simulink model "ctrl_PF"  (R2022b)
settings: Solver=FixedStepAuto  StartTime=0.0  StopTime=Tf  FixedStep=0.05  RelTol=1e-3
StopFcn:
  | save('testdata')
values from neighbouring files (symbols this model uses):
  Ba_0 = [0 0 0 0 0 0]    [run.m]    (also in testdata.mat)
  Bb = 4418825.3321    [testdata.mat]
  Bv_0 = [-5.14444 0 0 0 0 0]    [run.m]    (also in testdata.mat)
  Bx_0 = [-Cp(1,1) -Cp(2,1) Cp(3,1) 0 0 -pi]    [run.m]    (also in testdata.mat = [7.34788079488e-14 -400 -100 0 0 -3.14159265359])
  Cp = [x;y;z]    [run.m]    (also in testdata.mat = [-7.34788079488e-14 400 -100 -24.1026674607 399.273166418 -1)
  Cp_prime = Cp*Diff    [run.m]    (also in testdata.mat = [-4.77232815721 -0.143913049279 0 -4.75515990164 -0.42831409)
  d = 50    [run.m]    (also in testdata.mat)
  dA_BP1 = [0.00388591051125 0.00354364911083 0.00553040741788 0.00502167988714 0.0078585088908 0.00748424955325 0.0119232766011 0.0109054787122 0.0168329706434 0.016985509009 0.0156802934897 0.014556760782 ... (616 elements, 616x1)]    [testdata.mat]
  dA_BP2 = [0.00388594063171 0.00354357191533 0.00553040491113 0.00502170939051 0.00785855989083 0.00748435285791 0.0119232653011 0.0109054419481 0.0168329955973 0.0169854794658 0.015680230324 0.0145567225609 ... (616 elements, 616x1)]    [testdata.mat]
  dA_Hull = [0.896301676511 0.898896720864 0.884294141897 0.886832830172 0.870887902011 0.873360353662 0.856223658523 0.858613244346 0.840314828191 0.842595287849 0.823129385532 0.8253007603 ... (2914 elements, 2914x1)]    [testdata.mat]
  dA_PH = [0.00917454029683 0.00917454029683 0.00646521761836 0.00644666811643 0.011728531678 0.0107683420972 0.0165186720105 0.0100399866209 0.0121147162203 0.00917369783051 0.00917369783051 0.00646462373197 ... (550 elements, 550x1)]    [testdata.mat]
  dA_Sail = [0.08073747293 0.0655437895785 0.0678199581962 0.211496702297 0.185444652254 0.10949647106 0.0763960001413 0.0735864235671 0.0440728222699 0.281106392154 0.32735958292 0.104041938486 ... (564 elements, 564x1)]    [testdata.mat]
  dA_SProot = [0.0225345452169 0.0247277274893 0.0225345452169 0.0480467976325 0.0166447079844 0.0410754287554 0.0247277274893 0.0480467976325 0.0468898715351 0.0839833312794 0.0166447079844 0.0255016718 ... (904 elements, 904x1)]    [testdata.mat]
  dA_X1a = [0.0149621011817 0.0166706156701 0.0341149781095 0.0355915100668 0.0512235531199 0.0489176133683 0.0604458424392 0.0503279152264 0.0577124835488 0.0401555322121 0.044833653096 0.0251568218541 ... (200 elements, 200x1)]    [testdata.mat]
  dA_X1b = [0.0149621011817 0.0166706156701 0.0341149781095 0.0355915100668 0.0512235531199 0.0489176133683 0.0604458424392 0.0503279152264 0.0577124835488 0.0401555322121 0.044833653096 0.0251568218541 ... (200 elements, 200x1)]    [testdata.mat]
  dA_X2a = [0.0149620639393 0.0166705502855 0.0341150948266 0.0355913495849 0.051223110376 0.0489180393921 0.0604458270347 0.0503275686692 0.0577128112225 0.0401556683139 0.0448334591683 0.0251566482124 ... (200 elements, 200x1)]    [testdata.mat]
  dA_X2b = [0.0149620639393 0.0166705502855 0.0341150948266 0.0355913495849 0.051223110376 0.0489180393921 0.0604458270347 0.0503275686692 0.0577128112225 0.0401556683139 0.0448334591683 0.0251566482124 ... (200 elements, 200x1)]    [testdata.mat]
  dA_X3a = [0.0149621011817 0.0166706156701 0.0341149781095 0.0355915100668 0.0512235531199 0.0489176133683 0.0604458424392 0.0503279152264 0.0577124835488 0.0401555322121 0.044833653096 0.0251568218541 ... (200 elements, 200x1)]    [testdata.mat]
  dA_X3b = [0.0149621011817 0.0166706156701 0.0341149781095 0.0355915100668 0.0512235531199 0.0489176133683 0.0604458424392 0.0503279152264 0.0577124835488 0.0401555322121 0.044833653096 0.0251568218541 ... (200 elements, 200x1)]    [testdata.mat]
  dA_X4a = [0.0149621011817 0.0166706156701 0.0341149781095 0.0355915100668 0.0512235531199 0.0489176133683 0.0604458424392 0.0503279152264 0.0577124835488 0.0401555322121 0.044833653096 0.0251568218541 ... (200 elements, 200x1)]    [testdata.mat]
  dA_X4b = [0.0149621011817 0.0166706156701 0.0341149781095 0.0355915100668 0.0512235531199 0.0489176133683 0.0604458424392 0.0503279152264 0.0577124835488 0.0401555322121 0.044833653096 0.0251568218541 ... (200 elements, 200x1)]    [testdata.mat]
  Ixx = 52300000    [testdata.mat]
  Ixy = 0    [testdata.mat]
  Ixz = 0    [testdata.mat]
  Iyy = 1375000000    [testdata.mat]
  Iyz = 0    [testdata.mat]
  Izz = 1367000000    [testdata.mat]
  Ky = 1    [run.m]    (also in testdata.mat)
  Mb = 4418825.3321    [testdata.mat]
  n_BP1 = [-0.7747315 -0.03638153 -0.4095958 0 -0.1221389 0 -0.01670914 0 0.005209626 0 0.03404154 0 ... (1848 elements, 616x3)]    [testdata.mat]
  n_BP2 = [-0.774731517 -0.0363815315 -0.409595788 0 -0.122138903 0 -0.0167091396 0 0.00520962616 0 0.0340415388 0 ... (1848 elements, 616x3)]    [testdata.mat]
  n_Hull = [-3.334458e-05 -1.700098e-14 -3.354233e-05 -1.686235e-14 -3.289162e-05 -1.685701e-14 -3.291391e-05 -1.698144e-14 -3.338145e-05 -1.688959e-14 -3.29289e-05 -1.682536e-14 ... (8742 elements, 2914x3)]    [testdata.mat]
  n_PH = [0 0 0.01711651 0.01711627 0.2676807 0.2676804 0.7675173 0.7675174 0.9857236 0 0 0.01711456 ... (1650 elements, 550x3)]    [testdata.mat]
  n_Sail = [-0.05126832 -0.05168081 -0.0485872 -0.03288998 -0.03203588 -0.04435105 -0.04335441 -0.04419429 -0.05169604 0.01094904 0.01649325 -0.03825178 ... (1692 elements, 564x3)]    [testdata.mat]
  n_SProot = [-0.7837688 -0.7969784 -0.7837688 -0.79448 -0.280412 -0.3378876 -0.7969784 -0.79448 -0.7910827 -0.3483897 -0.280412 -0.2790298 ... (2712 elements, 904x3)]    [testdata.mat]
  n_X2a = [-0.283297986 -0.283136904 -0.283195704 -0.28313759 -0.2831586 -0.283137113 -0.28313911 -0.283136606 -0.283121586 -0.283136815 -0.283108413 -0.283138901 ... (600 elements, 200x3)]    [testdata.mat]
  n_X2b = [-0.283297986 -0.283136904 -0.283195704 -0.28313759 -0.2831586 -0.283137113 -0.28313911 -0.283136606 -0.283121586 -0.283136815 -0.283108413 -0.283138901 ... (600 elements, 200x3)]    [testdata.mat]
  n_X3a = [-0.283298 -0.2831369 -0.2831957 -0.2831376 -0.2831586 -0.2831371 -0.2831391 -0.2831366 -0.2831216 -0.2831368 -0.2831084 -0.2831389 ... (600 elements, 200x3)]    [testdata.mat]
  n_X4a = [-0.283298 -0.2831369 -0.2831957 -0.2831376 -0.2831586 -0.2831371 -0.2831391 -0.2831366 -0.2831216 -0.2831368 -0.2831084 -0.2831389 ... (600 elements, 200x3)]    [testdata.mat]
  n_X4b = [-0.283298 -0.2831369 -0.2831957 -0.2831376 -0.2831586 -0.2831371 -0.2831391 -0.2831366 -0.2831216 -0.2831368 -0.2831084 -0.2831389 ... (600 elements, 200x3)]    [testdata.mat]
  nt_BP1 = 616    [testdata.mat]
  nt_BP2 = 616    [testdata.mat]
  nt_Hull = 2914    [testdata.mat]
  nt_PH = 550    [testdata.mat]
  nt_Sail = 564    [testdata.mat]
  nt_SProot = 904    [testdata.mat]
  nt_X1a = 200    [testdata.mat]
  nt_X1b = 200    [testdata.mat]
  nt_X2a = 200    [testdata.mat]
  nt_X2b = 200    [testdata.mat]
  nt_X3a = 200    [testdata.mat]
  nt_X3b = 200    [testdata.mat]
  nt_X4a = 200    [testdata.mat]
  nt_X4b = 200    [testdata.mat]
  Seastate = 0    [run.m]    (also in testdata.mat)
  Tf = 500    [run.m]    (also in testdata.mat)
  v_ref = Bv_0(1)    [run.m]    (also in testdata.mat = -5.14444)
  vt1_BP1 = [-11.0524049722 -10.9924120522 -10.9924120522 -10.8819663922 -10.8819663922 -10.7297166322 -10.7297166322 -10.5070632922 -10.5070632922 -10.1807245522 -10.1807245522 -9.8815181122 ... (1848 elements, 616x3)]    [testdata.mat]
  vt1_BP2 = [-11.0524048318 -10.9924111396 -10.9924111396 -10.8819658306 -10.8819658306 -10.7297157898 -10.7297157898 -10.5070637134 -10.5070637134 -10.1807238502 -10.1807238502 -9.8815188844 ... (1848 elements, 616x3)]    [testdata.mat]
  vt1_Hull = [3.5122487678 3.7304022878 5.2621803278 5.4863499878 6.9866994878 7.2167238278 8.6832650078 8.9189474678 10.3493567078 10.5904445678 11.9823842078 12.2286247478 ... (8742 elements, 2914x3)]    [testdata.mat]
  vt1_PH = [37.3342788278 37.3342788278 37.4268866678 37.4268866678 37.5892452278 37.5892452278 37.7549453078 37.7549453078 37.8074619278 37.3342788278 37.3342788278 37.4268866678 ... (1650 elements, 550x3)]    [testdata.mat]
  vt1_Sail = [-12.4909433722 -12.1578443722 -12.0399645322 -11.2138368922 -10.6240515922 -11.5111900522 -11.9364967522 -11.6561249722 -12.4909433722 -7.5732648922 -6.8453119522 -11.1890071522 ... (1692 elements, 564x3)]    [testdata.mat]
  vt1_SProot = [29.2099766678 29.1371231078 29.0494854278 29.2099766678 29.2862630078 29.4526510478 29.0494854278 29.1261368078 29.3369263478 29.5706712878 29.0494854278 29.3857364078 ... (2712 elements, 904x3)]    [testdata.mat]
  vt1_X1a = [29.3961751478 29.4776282078 29.4776282078 29.7060309278 29.7060309278 30.0693861278 30.0693861278 30.5458756478 30.5458756478 31.0830460478 31.0830460478 31.6023926678 ... (600 elements, 200x3)]    [testdata.mat]
  vt1_X1b = [29.6638337078 29.6638337078 29.9620713878 29.9620713878 30.3181187678 30.3181187678 30.7116389078 30.7116389078 31.1104380878 31.1104380878 31.4810519678 31.4810519678 ... (600 elements, 200x3)]    [testdata.mat]
  vt1_X2a = [29.3961767624 29.4776272952 29.4776272952 29.7060326828 29.7060326828 30.0693842324 30.0693842324 30.5458736822 30.5458736822 31.083047171 31.083047171 31.6023916148 ... (600 elements, 200x3)]    [testdata.mat]
  vt1_X2b = [29.6638345502 29.6638345502 29.9620708964 29.9620708964 30.3181168022 30.3181168022 30.7116409436 30.7116409436 31.1104372454 31.1104372454 31.4810526698 31.4810526698 ... (600 elements, 200x3)]    [testdata.mat]
  vt1_X3a = [29.3961751478 29.4776282078 29.4776282078 29.7060309278 29.7060309278 30.0693861278 30.0693861278 30.5458756478 30.5458756478 31.0830460478 31.0830460478 31.6023926678 ... (600 elements, 200x3)]    [testdata.mat]
  vt1_X3b = [29.6638337078 29.6638337078 29.9620713878 29.9620713878 30.3181187678 30.3181187678 30.7116389078 30.7116389078 31.1104380878 31.1104380878 31.4810519678 31.4810519678 ... (600 elements, 200x3)]    [testdata.mat]
  vt1_X4a = [29.6638337078 29.6638337078 29.9620713878 29.9620713878 30.3181187678 30.3181187678 30.7116389078 30.7116389078 31.1104380878 31.1104380878 31.4810519678 31.4810519678 ... (600 elements, 200x3)]    [testdata.mat]
  vt1_X4b = [29.3961751478 29.4776282078 29.4776282078 29.7060309278 29.7060309278 30.0693861278 30.0693861278 30.5458756478 30.5458756478 31.0830460478 31.0830460478 31.6023926678 ... (600 elements, 200x3)]    [testdata.mat]
  vt2_BP1 = [-10.9924120522 -10.9494777322 -10.8819663922 -10.8505308322 -10.7297166322 -10.7112259522 -10.5070632922 -10.4997203722 -10.1807245522 -10.1757543922 -9.8815181122 -9.8813004922 ... (1848 elements, 616x3)]    [testdata.mat]
  vt2_BP2 = [-11.0294626294 -11.0294626294 -10.9494786448 -10.9494786448 -10.8505316746 -10.8505316746 -10.7112256012 -10.7112256012 -10.499720302 -10.499720302 -10.1757550942 -10.1757550942 ... (1848 elements, 616x3)]    [testdata.mat]
  vt2_Hull = [1.9517168078 1.9517168078 3.7304022878 3.7304022878 5.4863499878 5.4863499878 7.2167238278 7.2167238278 8.9189474678 8.9189474678 10.5904445678 10.5904445678 ... (8742 elements, 2914x3)]    [testdata.mat]
  vt2_PH = [37.2028433678 37.2028433678 37.3342788278 37.4268866678 37.4268866678 37.5892452278 37.5892452278 37.7549453078 37.7549453078 37.2028433678 37.2028433678 37.3342788278 ... (1650 elements, 550x3)]    [testdata.mat]
  vt2_Sail = [-12.0399645322 -12.0399645322 -11.9364967522 -10.7084881522 -10.7084881522 -12.0399645322 -12.0399645322 -11.9364967522 -12.3734566522 -7.7110323922 -7.7110323922 -11.6561249722 ... (1692 elements, 564x3)]    [testdata.mat]
  vt2_SProot = [29.0494854278 29.0494854278 29.2099766678 29.1261368078 29.0494854278 29.1371231078 29.1371231078 29.2099766678 29.1261368078 29.2099766678 29.2862630078 29.2862630078 ... (2712 elements, 904x3)]    [testdata.mat]
  vt2_X1a = [29.4776282078 29.9620713878 29.7060309278 30.3181187678 30.0693861278 30.7116389078 30.5458756478 31.1104380878 31.0830460478 31.4810519678 31.6023926678 31.7970362078 ... (600 elements, 200x3)]    [testdata.mat]
  vt2_X1b = [29.4776282078 29.9620713878 29.7060309278 30.3181187678 30.0693861278 30.7116389078 30.5458756478 31.1104380878 31.0830460478 31.4810519678 31.6023926678 31.7970362078 ... (600 elements, 200x3)]    [testdata.mat]
  vt2_X2a = [29.6638345502 29.6638345502 29.9620708964 29.9620708964 30.3181168022 30.3181168022 30.7116409436 30.7116409436 31.1104372454 31.1104372454 31.4810526698 31.4810526698 ... (600 elements, 200x3)]    [testdata.mat]
  vt2_X2b = [29.3961767624 29.4776272952 29.4776272952 29.7060326828 29.7060326828 30.0693842324 30.0693842324 30.5458736822 30.5458736822 31.083047171 31.083047171 31.6023916148 ... (600 elements, 200x3)]    [testdata.mat]
  vt2_X3a = [29.4776282078 29.9620713878 29.7060309278 30.3181187678 30.0693861278 30.7116389078 30.5458756478 31.1104380878 31.0830460478 31.4810519678 31.6023926678 31.7970362078 ... (600 elements, 200x3)]    [testdata.mat]
  vt2_X3b = [29.4776282078 29.9620713878 29.7060309278 30.3181187678 30.0693861278 30.7116389078 30.5458756478 31.1104380878 31.0830460478 31.4810519678 31.6023926678 31.7970362078 ... (600 elements, 200x3)]    [testdata.mat]
  vt2_X4a = [29.4776282078 29.9620713878 29.7060309278 30.3181187678 30.0693861278 30.7116389078 30.5458756478 31.1104380878 31.0830460478 31.4810519678 31.6023926678 31.7970362078 ... (600 elements, 200x3)]    [testdata.mat]
  vt2_X4b = [29.4776282078 29.9620713878 29.7060309278 30.3181187678 30.0693861278 30.7116389078 30.5458756478 31.1104380878 31.0830460478 31.4810519678 31.6023926678 31.7970362078 ... (600 elements, 200x3)]    [testdata.mat]
  vt3_BP1 = [-11.0294636122 -11.0294636122 -10.9494777322 -10.9494777322 -10.8505308322 -10.8505308322 -10.7112259522 -10.7112259522 -10.4997203722 -10.4997203722 -10.1757543922 -10.1757543922 ... (1848 elements, 616x3)]    [testdata.mat]
  vt3_BP2 = [-10.9924111396 -10.9494786448 -10.8819658306 -10.8505316746 -10.7297157898 -10.7112256012 -10.5070637134 -10.499720302 -10.1807238502 -10.1757550942 -9.8815188844 -9.8813013346 ... (1848 elements, 616x3)]    [testdata.mat]
  vt3_Hull = [1.7397198278 3.5122487678 3.5122487678 5.2621803278 5.2621803278 6.9866994878 6.9866994878 8.6832650078 8.6832650078 10.3493567078 10.3493567078 11.9823842078 ... (8742 elements, 2914x3)]    [testdata.mat]
  vt3_PH = [37.2028433678 37.3342788278 37.3342788278 37.3342788278 37.4268866678 37.4268866678 37.5892452278 37.5892452278 37.7549453078 37.2028433678 37.3342788278 37.3342788278 ... (1650 elements, 550x3)]    [testdata.mat]
  vt3_Sail = [-12.3734566522 -12.4909433722 -12.3734566522 -11.5111900522 -11.2138368922 -11.7698559922 -11.5111900522 -11.5111900522 -12.1578443722 -8.3109054322 -7.5732648922 -11.5111900522 ... (1692 elements, 564x3)]    [testdata.mat]
  vt3_SProot = [29.1261368078 29.2099766678 29.1261368078 29.3369263478 29.1371231078 29.2099766678 29.2099766678 29.3369263478 29.2548344678 29.3369263478 29.1371231078 29.1371231078 ... (2712 elements, 904x3)]    [testdata.mat]
  vt3_X1a = [29.6638337078 29.6638337078 29.9620713878 29.9620713878 30.3181187678 30.3181187678 30.7116389078 30.7116389078 31.1104380878 31.1104380878 31.4810519678 31.4810519678 ... (600 elements, 200x3)]    [testdata.mat]
  vt3_X1b = [29.3961751478 29.4776282078 29.4776282078 29.7060309278 29.7060309278 30.0693861278 30.0693861278 30.5458756478 30.5458756478 31.0830460478 31.0830460478 31.6023926678 ... (600 elements, 200x3)]    [testdata.mat]
  vt3_X2a = [29.4776272952 29.9620708964 29.7060326828 30.3181168022 30.0693842324 30.7116409436 30.5458736822 31.1104372454 31.083047171 31.4810526698 31.6023916148 31.7970343826 ... (600 elements, 200x3)]    [testdata.mat]
  vt3_X2b = [29.4776272952 29.9620708964 29.7060326828 30.3181168022 30.0693842324 30.7116409436 30.5458736822 31.1104372454 31.083047171 31.4810526698 31.6023916148 31.7970343826 ... (600 elements, 200x3)]    [testdata.mat]
  vt3_X3a = [29.6638337078 29.6638337078 29.9620713878 29.9620713878 30.3181187678 30.3181187678 30.7116389078 30.7116389078 31.1104380878 31.1104380878 31.4810519678 31.4810519678 ... (600 elements, 200x3)]    [testdata.mat]
  vt3_X3b = [29.3961751478 29.4776282078 29.4776282078 29.7060309278 29.7060309278 30.0693861278 30.0693861278 30.5458756478 30.5458756478 31.0830460478 31.0830460478 31.6023926678 ... (600 elements, 200x3)]    [testdata.mat]
  vt3_X4a = [29.3961751478 29.4776282078 29.4776282078 29.7060309278 29.7060309278 30.0693861278 30.0693861278 30.5458756478 30.5458756478 31.0830460478 31.0830460478 31.6023926678 ... (600 elements, 200x3)]    [testdata.mat]
  vt3_X4b = [29.6638337078 29.6638337078 29.9620713878 29.9620713878 30.3181187678 30.3181187678 30.7116389078 30.7116389078 31.1104380878 31.1104380878 31.4810519678 31.4810519678 ... (600 elements, 200x3)]    [testdata.mat]
  Xb = 0    [testdata.mat]
  Xcg = [32.3287332922 0 0]    [testdata.mat]
  Xg = 0    [testdata.mat]
  Yb = 0    [testdata.mat]
  Yg = 0    [testdata.mat]
  Zb = 0.4406    [testdata.mat]
  Zg = 0    [testdata.mat]
undefined symbols (not defined in the file or in its folder): Cpv
libraries: simulink x8, sharedtransform x2, dspmathops x2
(part 2 of 8)

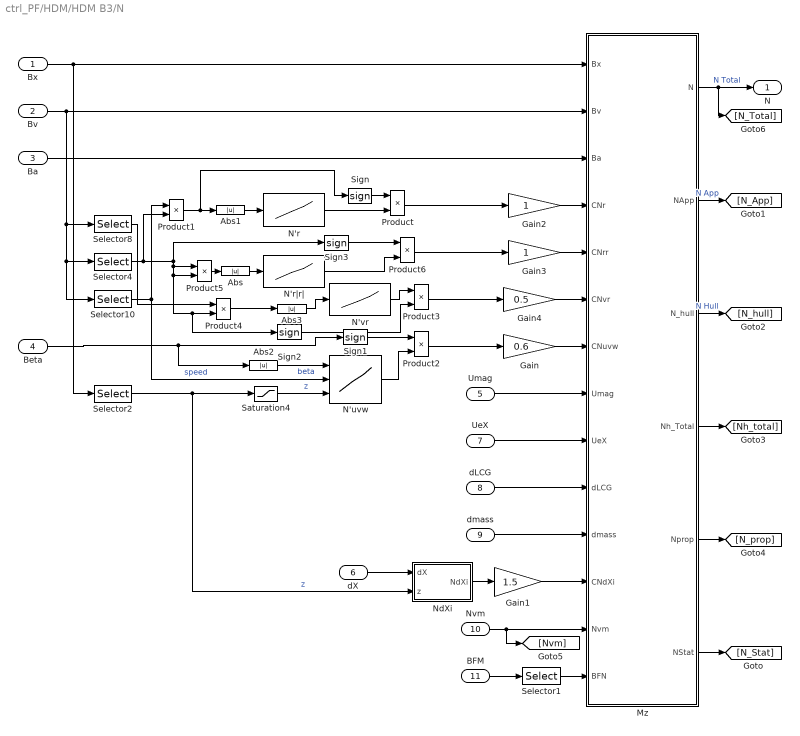
== system ctrl_PF/HDM/HDM B3/N ==
  Bx : Inport
  Bv : Inport  Port=2
  Ba : Inport  Port=3
  Beta : Inport  Port=4
  Umag : Inport  Port=5
  dX : Inport  Port=6
  UeX : Inport  Port=7
  dLCG : Inport  Port=8
  dmass : Inport  Port=9
  Nvm : Inport  Port=10
  BFM : Inport  Port=11
  Abs{,1..3} (4 alike) : Abs  SaturateOnIntegerOverflow=off
  Gain : Gain  Gain=0.6
  Gain1 : Gain  Gain=1.5
  Gain2 : Gain
  Gain3 : Gain
  Gain4 : Gain  Gain=0.5
  Mz : MATLAB Function  TreatAsAtomicUnit=on
  N'r : Lookup_n-D  NumberOfTableDimensions=1  BreakpointsForDimension1=|  Table=|  InternalRulePriority=Speed  RndMeth=Simplest
      BreakpointsForDimension1=|
      | [0.03999989
      | 0.079999993
      | 0.11999963
      | 0.15999956]
      Table=|
      | [-4.0344E-04
      | -8.1402E-04
      | -1.2116E-03
      | -1.6125E-03]
  N'r|r| : Lookup_n-D  NumberOfTableDimensions=1  BreakpointsForDimension1=|  Table=|  InternalRulePriority=Speed  RndMeth=Simplest
      BreakpointsForDimension1=|
      | [0.0001
      | 0.0003
      | 0.0006
      | 0.0009
      | 0.0012
      | 0.0015
      | ]
      Table=|
      | [1.93E-01
      | 6.44E-02
      | 3.19E-02
      | 2.11E-02
      | 1.64E-02
      | 1.34E-02
      | ]
  N'uvw : Lookup_n-D  NumberOfTableDimensions=3  BreakpointsForDimension1=|  BreakpointsForDimension2=|  BreakpointsForDimension3=|  Table=|  InternalRulePriority=Speed  RndMeth=Simplest
      BreakpointsForDimension1=|
      | [0
      | 4
      | 8
      | 12]
      BreakpointsForDimension2=|
      | [-5.1444E+00
      | -3.0866E+00
      | -1.5433E+00
      | ]
      Table=|
      | reshape([0.0000000E+00
      | 1.1975814E-03
      | 2.7970643E-03
      | 4.1308534E-03
      | 0.0000000E+00
      | 1.2111628E-03
      | 2.9207146E-03
      | 4.1207837E-03
      | 0.0000000E+00
      | 1.4959851E-03
      | 2.9486406E-03
      | 4.1213058E-03
      | 0.0000000E+00
      | 1.4879743E-03
      | 2.9975710E-03
      | 4.2577903E-03
      | 0.0000000E+00
      | 1.4933232E-03
      | 3.0017417E-03
      | 4.2334501E-03
      | 0.0000000E+00
      | 1.5365285E-03
      | 3.0446384E-03
      | 4.4091424E-03
      | 0.0000000E+00
      | 1.5329300E-03
      | 3.0664177E-03
      | 4.3937198E-03
      | 0.0000000E+00
      | 1.5274021E-03
      | 3.0742094E-03
      | 4.3066710E-03
      | 0.0000000E+00
      | 1.5692494E-03
      | 3.1052278E-03
      | 4.3211963E-03
      | 0.0000000E+00
      | 1.5996020E-03
      | 3.2227652E-03
      | 4.5425478E-03
      | 0.0000000E+00
      | 1.5650123E-03
      | 3.1236229E-03
      | 4.4022471E-03
      | 0.0000000E+00
      | 1.6041810E-03
      | 3.1241151E-03
      | 4.4103656E-03],[4,3,4])
      BreakpointsForDimension3=|
      | [-35.0624 -18.3724 -15.3724 -13.8724
      | ]
      settings: InputPortMap=u0,u1,u2
  N'vr : Lookup_n-D  NumberOfTableDimensions=1  BreakpointsForDimension1=|  Table=|  InternalRulePriority=Speed  RndMeth=Simplest
      BreakpointsForDimension1=|
      | [0
      | 0.051444
      | 0.102888
      | 0.205776
      | 0.411552]
      Table=|
      | [0.0000E+00
      | -1.9921E-03
      | -9.2025E-03
      | -3.2154E-02
      | -1.3255E-01]
  NdXi : Subsystem
  Product{,1..6} (7 alike) : Product
  Saturation4 : Saturate  UpperLimit=-13.8724  LowerLimit=-35.0624
  Selector1 : Selector  InputPortWidth=6  IndexOptions=Index vector (dialog)  Indices=6  OutputSizes=1
  Selector10 : Selector  InputPortWidth=6  IndexOptions=Index vector (dialog)  Indices=1  OutputSizes=1
  Selector2 : Selector  InputPortWidth=6  IndexOptions=Index vector (dialog)  Indices=3  OutputSizes=1
  Selector4 : Selector  InputPortWidth=6  IndexOptions=Index vector (dialog)  Indices=6  OutputSizes=1
  Selector8 : Selector  InputPortWidth=6  IndexOptions=Index vector (dialog)  Indices=2  OutputSizes=1
  Sign{,1..3} (4 alike) : Signum
  N : Outport
  wires:
  Mz/5(Nprop) -> [N_prop]
  Mz/4(Nh_Total) -> [Nh_total]
  Mz/3(N_hull) -> [N_hull]  "N Hull"
  Mz/2(NApp) -> [N_App]  "N App"
  Abs/1 -> N'r|r|/1
  Sign3/1 -> Product6/1
  Product6/1 -> Gain3/1
  Sign2/1 -> Product3/2
  N'vr/1 -> Product3/1
  Abs3/1 -> N'vr/1
  Saturation4/1 -> N'uvw/3  "z"
  Gain4/1 -> Mz/6(CNvr)
  Gain3/1 -> Mz/5(CNrr)
  Gain2/1 -> Mz/4(CNr)
  Mz/6(NStat) -> [N_Stat]
  Selector1/1 -> Mz/14(BFN)
  BFM/1 -> Selector1/1
  Nvm/1 -> [Nvm], Mz/13(Nvm)
  Gain1/1 -> Mz/12(CNdXi)
  NdXi/1(NdXi) -> Gain1/1
  Gain/1 -> Mz/7(CNuvw)
  Product2/1 -> Gain/1
  Sign1/1 -> Product2/1
  Abs2/1 -> N'uvw/1  "beta"
  Product/1 -> Gain2/1
  Sign/1 -> Product/1
  Abs1/1 -> N'r/1
  Product1/1 -> Abs1/1, Sign/1
  N'uvw/1 -> Product2/2
  Selector2/1 -> Saturation4/1, NdXi/2(z)  "z"
  Mz/1(N) -> [N_Total], N/1  "N Total"
  Product3/1 -> Gain4/1
  Product5/1 -> Abs/1
  Selector4/1 -> Product1/2, Sign3/1, Product5/2, Sign2/1, Product4/2, Product5/1
  Selector8/1 -> Product4/1
  Product4/1 -> Abs3/1
  N'r|r|/1 -> Product6/2
  N'r/1 -> Product/2
  dX/1 -> NdXi/1(dX)
  dmass/1 -> Mz/11(dmass)
  dLCG/1 -> Mz/10(dLCG)
  Umag/1 -> Mz/8(Umag)
  Beta/1 -> Sign1/1, Abs2/1
  UeX/1 -> Mz/9(UeX)
  Ba/1 -> Mz/3(Ba)
  Selector10/1 -> Product1/1, N'uvw/2  "speed"
  Bx/1 -> Mz/1(Bx), Selector2/1
  Bv/1 -> Mz/2(Bv), Selector8/1, Selector4/1, Selector10/1

== system ctrl_PF/HDM/HDM B3/Thrust & Torque ==
  In1 : Inport
  In2 : Inport  Port=2
  n_0 : Inport  Port=3
  Gain20 : Gain  Gain=-1
  Saturation5 : Saturate  UpperLimit=-13.8724  LowerLimit=-36.3724
  Saturation7 : Saturate  UpperLimit=-1.54333333  LowerLimit=-5.14444
  "Thrust Deduction, 25m1" : Lookup_n-D  BreakpointsForDimension1=|  BreakpointsForDimension2=[-5.14444 -3.086664 -1.543332]  Table=|  InternalRulePriority=Speed  RndMeth=Simplest
      BreakpointsForDimension1=|
      | [-36.3724
      | -18.3724
      | -15.3724
      | -13.8724]
      Table=|
      | reshape([0.245958
      | 0.251311246
      | 0.25251
      | 0.251322
      | 0.2444134
      | 0.2498597
      | 0.2509219
      | 0.2498992
      | 0.2496
      | 0.2594532
      | 0.257802
      | 0.2475762],[4,3])
      settings: InputPortMap=u0,u1
  Tprop : MATLAB Function  TreatAsAtomicUnit=on
  Tprop1 : Outport
  Qprop : Outport  Port=2
  wires:
  n_0/1 -> Tprop/3(n_0)
  Saturation7/1 -> "Thrust Deduction, 25m1"/2
  Tprop/2(Qprop) -> Qprop/1
  Gain20/1 -> Tprop/1(speed)
  Saturation5/1 -> "Thrust Deduction, 25m1"/1
  "Thrust Deduction, 25m1"/1 -> Tprop/2(Td)
  Tprop/1(Tprop) -> Tprop1/1
  In2/1 -> Saturation7/1
  In1/1 -> Gain20/1, Saturation5/1

== system ctrl_PF/HDM/HDM B3/Wave, Virtual Mass and Hydrostatic ==
  Bx_earth : Inport
  Bv_ship : Inport  Port=2
  SeaState : Inport  Port=3
  dLCG : Inport  Port=4
  dX_CTRL : Inport  Port=5
  Add : Sum  Inputs=+-
  CG : Constant  Value=Xcg
  CGi : Constant  Value=|
      | [5.0784E+00	0.0000E+00	8.0728E-03;
      | 1.1013E+01	0.0000E+00	2.5384E-01;
      | 1.7302E+01	0.0000E+00	3.0728E-01;
      | 2.5741E+01	0.0000E+00	4.1417E-01;
      | 3.4688E+01	0.0000E+00	4.1585E-01;
      | 4.2324E+01	0.0000E+00	3.2444E-01;
      | 4.9992E+01	0.0000E+00	3.3454E-01;
      | 5.7427E+01	0.0000E+00	1.7420E-02;
      | 6.3078E+01	0.0000E+00	1.8824E-02;
      | 6.6703E+01	0.0000E+00	1.1340E-02;
      | 2.5141E+01	0.0000E+00	8.6491E+00;
      | 2.1732E+01	0.0000E+00	9.7273E+00;
      | 6.3166E+01	0.0000E+00	-4.0823E-17;
      | 2.2043E+01	0.0000E+00	9.7261E+00;
      | 6.3451E+01	0.0000E+00	-6.2238E-17;
      | ]
  Cvm*dm : Constant  Value=|
      | [8.4658E+04	1.7229E+05	1.6487E+05
      | 2.3551E+04	4.3394E+05	3.6176E+05
      | 1.1585E+03	5.9767E+05	4.2996E+05
      | 1.4123E+02	1.1354E+06	6.5606E+05
      | 9.1503E+01	6.9712E+05	5.1688E+05
      | 9.6110E+01	6.7201E+05	5.1905E+05
      | 1.2163E+04	5.7818E+05	4.7547E+05
      | 3.7219E+04	3.4697E+05	3.3508E+05
      | 1.9318E+04	7.7284E+04	7.6560E+04
      | 1.5368E+04	2.6375E+04	2.6268E+04
      | 1.8312E+04	4.5870E+05	5.1108E+04
      | 3.1859E+02	1.2645E+04	3.4886E+02
      | 3.0285E+03	4.4945E+04	4.4489E+04
      | 7.9160E+02	8.8963E+02	1.3306E+04
      | 1.2115E+03	3.9547E+04	3.9205E+04
      | ]
  Demux : Demux  Outputs=3
  Demux1 : Demux  Outputs=3
  Derivative1 : Derivative
  MATLAB Function : MATLAB Function  TreatAsAtomicUnit=on
  Wave Particle Motions : Subsystem
  beta_wave : Constant  Value=0
  phi_wave : Constant  Value=0
  Xvm : Outport
  Yvm : Outport  Port=2
  Zvm : Outport  Port=3
  Kvm : Outport  Port=4
  Mvm : Outport  Port=5
  Nvm : Outport  Port=6
  uwsXi : Outport  Port=7
  uwsCG : Outport  Port=8
  B_FM : Outport  Port=9
  wires:
  beta_wave/1 -> Wave Particle Motions/9(beta_wave)
  phi_wave/1 -> Wave Particle Motions/8(phi_wave)
  dX_CTRL/1 -> Wave Particle Motions/7(dX_CTRL)
  Cvm*dm/1 -> MATLAB Function/2(cvm)
  Wave Particle Motions/5(B_FM) -> B_FM/1
  Derivative1/1 -> MATLAB Function/3(Awrs)  "d/dt(aw-ar)"
  Add/1 -> Derivative1/1
  Wave Particle Motions/3(urs) -> Add/2
  Wave Particle Motions/2(uws) -> Add/1
  Wave Particle Motions/6(uwsCG) -> uwsCG/1
  Wave Particle Motions/4(uwXis) -> uwsXi/1
  Demux1/3 -> Nvm/1
  Demux1/1 -> Kvm/1
  Demux1/2 -> Mvm/1
  Demux/3 -> Zvm/1
  Demux/2 -> Yvm/1
  Demux/1 -> Xvm/1
  MATLAB Function/2(Mvm) -> Demux1/1  "Mvm"
  MATLAB Function/1(Fvm) -> Demux/1  "Fvm"
  Bv_ship/1 -> Wave Particle Motions/1(U_ship)
  dLCG/1 -> Wave Particle Motions/6(dLCG)
  SeaState/1 -> Wave Particle Motions/5(SeaState)
  Wave Particle Motions/1(Rs) -> MATLAB Function/1(Rs)
  CG/1 -> Wave Particle Motions/4(CG)
  CGi/1 -> Wave Particle Motions/3(CGi)
  Bx_earth/1 -> Wave Particle Motions/2(X_earth)

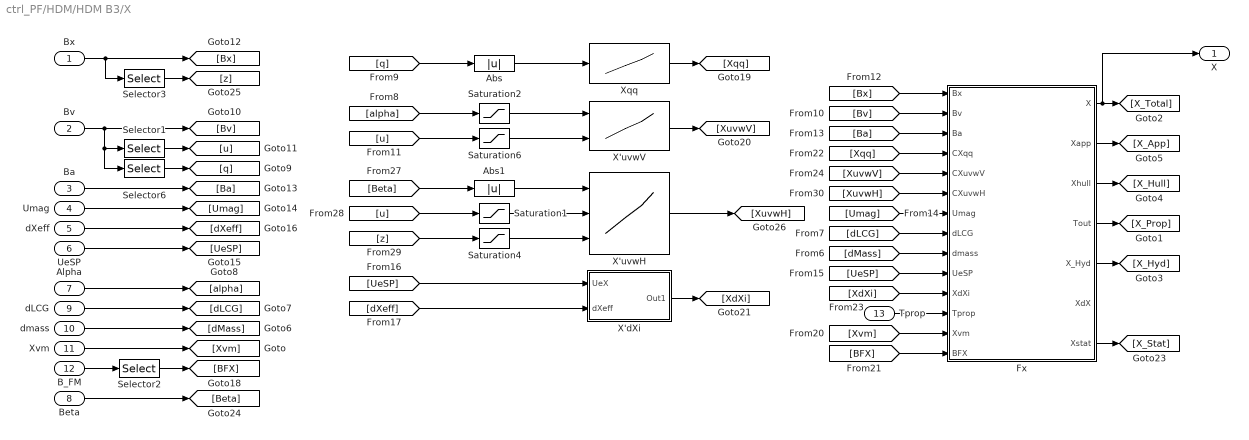
== system ctrl_PF/HDM/HDM B3/X ==
  Bx : Inport
  Bv : Inport  Port=2
  Ba : Inport  Port=3
  Umag : Inport  Port=4
  dXeff : Inport  Port=5
  UeSP : Inport  Port=6
  Alpha : Inport  Port=7
  Beta : Inport  Port=8
  dLCG : Inport  Port=9
  dmass : Inport  Port=10
  Xvm : Inport  Port=11
  B_FM : Inport  Port=12
  Tprop : Inport  Port=13
  Abs : Abs  SaturateOnIntegerOverflow=off
  Abs1 : Abs  SaturateOnIntegerOverflow=off
  Fx : MATLAB Function  TreatAsAtomicUnit=on
  Saturation1 : Saturate  UpperLimit=-1.543332  LowerLimit=-5.14444
  Saturation2 : Saturate  UpperLimit=30  LowerLimit=-30
  Saturation4 : Saturate  UpperLimit=-13.8724  LowerLimit=-35.0624
  Saturation6 : Saturate  UpperLimit=-1.543332  LowerLimit=-5.14444
  Selector1 : Selector  InputPortWidth=6  IndexOptions=Index vector (dialog)  Indices=1  OutputSizes=1
  Selector2 : Selector  InputPortWidth=6  IndexOptions=Index vector (dialog)  Indices=1  OutputSizes=1
  Selector3 : Selector  InputPortWidth=6  IndexOptions=Index vector (dialog)  Indices=3  OutputSizes=1
  Selector6 : Selector  InputPortWidth=6  IndexOptions=Index vector (dialog)  Indices=5  OutputSizes=1
  X'dXi : Subsystem
  X'uvwH : Lookup_n-D  NumberOfTableDimensions=3  BreakpointsForDimension1=|  BreakpointsForDimension2=|  BreakpointsForDimension3=|  Table=|  InternalRulePriority=Speed  RndMeth=Simplest
      BreakpointsForDimension1=|
      | [0
      | 4
      | 8
      | 12]
      BreakpointsForDimension2=|
      | [-5.1444
      | -3.08664
      | -1.54332]
      Table=|
      | reshape([0.0000000E+00
      | 8.7490400E-05
      | -4.2970032E-04
      | -8.6882993E-04
      | 0.0000000E+00
      | 9.2255510E-05
      | -3.6462757E-04
      | -8.6516720E-04
      | 0.0000000E+00
      | -8.0508235E-05
      | -3.3610820E-04
      | -9.1603355E-04
      | 0.0000000E+00
      | -9.0915847E-05
      | -3.9252667E-04
      | -9.2068441E-04
      | 0.0000000E+00
      | -1.0407599E-04
      | -3.8836462E-04
      | -9.1865822E-04
      | 0.0000000E+00
      | -8.4723950E-05
      | -3.5324770E-04
      | -9.7126434E-04
      | 0.0000000E+00
      | -9.3766627E-05
      | -4.1342843E-04
      | -9.4161914E-04
      | 0.0000000E+00
      | -1.0916277E-04
      | -4.0683220E-04
      | -9.6707684E-04
      | 0.0000000E+00
      | -8.8664811E-05
      | -3.7605406E-04
      | -9.4194453E-04
      | 0.0000000E+00
      | -9.2876985E-05
      | -4.0365964E-04
      | -9.3239814E-04
      | 0.0000000E+00
      | -1.1414747E-04
      | -4.4323139E-04
      | -1.0049645E-03
      | 0.0000000E+00
      | -9.4615234E-05
      | -4.9251136E-04
      | -9.8471513E-04],[4,3,4])
      BreakpointsForDimension3=|
      | [-35.0624 -18.3724 -15.3724 -13.8724
      | ]
      settings: InputPortMap=u0,u1,u2
  X'uvwV : Lookup_n-D  BreakpointsForDimension1=|  BreakpointsForDimension2=|  Table=|  InternalRulePriority=Speed  RndMeth=Simplest
      BreakpointsForDimension1=|
      | [-12
      | -8
      | -4
      | 0
      | 4
      | 8
      | 12]
      BreakpointsForDimension2=|
      | [-5.1444
      | -3.08664
      | -1.54332]
      Table=|
      | reshape([8.5556500E-04
      | 9.0045500E-04
      | 9.7379500E-04
      | 1.0292250E-03
      | 1.0286950E-03
      | 9.7963500E-04
      | 1.0147450E-03
      | 9.0637500E-04
      | 9.3710500E-04
      | 1.0133950E-03
      | 1.0723650E-03
      | 1.0693650E-03
      | 1.0284650E-03
      | 1.1084650E-03
      | 9.8653120E-04
      | 9.9350120E-04
      | 1.0534412E-03
      | 1.1098412E-03
      | 1.1115412E-03
      | 1.0836412E-03
      | 1.1582412E-03],[7,3])
      settings: InputPortMap=u0,u1
  Xqq : Lookup_n-D  NumberOfTableDimensions=1  BreakpointsForDimension1=|  Table=|  InternalRulePriority=Speed  RndMeth=Simplest
      BreakpointsForDimension1=|
      | [-0.02
      | -0.015
      | -0.012958963
      | -0.009719222
      | -0.006479482
      | -0.003239741
      | -0.00161987
      | -0.000647948
      | 0.000647948
      | 0.00161987
      | 0.003239741
      | 0.006479482
      | 0.009719222
      | 0.012958963
      | 0.015
      | 0.02
      | ]
      Table=|
      | [1.5581E-04
      | 1.1369E-04
      | 2.0348E-04
      | 4.5268E-04
      | 3.8456E-04
      | 9.9241E-05
      | 3.8998E-04
      | 9.1300E-05
      | -3.1574E-04
      | -7.9139E-05
      | -9.0517E-04
      | -4.4764E-04
      | -5.9612E-04
      | -5.5873E-04
      | -5.9343E-04
      | -5.5869E-04
      | ]
  X : Outport
  wires:
  [XuvwH] -> Fx/6(CXuvwH)
  X'uvwH/1 -> [XuvwH]
  Saturation4/1 -> X'uvwH/3
  [z] -> Saturation4/1
  Selector3/1 -> [z]
  Saturation1/1 -> X'uvwH/2
  [u] -> Saturation1/1
  [Beta] -> Abs1/1
  Abs1/1 -> X'uvwH/1
  Beta/1 -> [Beta]
  Tprop/1 -> Fx/12(Tprop)
  [XuvwV] -> Fx/5(CXuvwV)
  [XdXi] -> Fx/11(XdXi)
  X'dXi/1(Out1) -> [XdXi]
  X'uvwV/1 -> [XuvwV]
  Xqq/1 -> [Xqq]
  [Xqq] -> Fx/4(CXqq)
  [BFX] -> Fx/14(BFX)
  Selector2/1 -> [BFX]
  [Xvm] -> Fx/13(Xvm)
  Xvm/1 -> [Xvm]
  dXeff/1 -> [dXeff]
  [dXeff] -> X'dXi/2(dXeff)
  [UeSP] -> X'dXi/1(UeX)
  UeSP/1 -> [UeSP]
  [UeSP] -> Fx/10(UeSP)
  Umag/1 -> [Umag]
  [Umag] -> Fx/7(Umag)
  Ba/1 -> [Ba]
  [Ba] -> Fx/3(Ba)
  Bx/1 -> Selector3/1, [Bx]
  [Bx] -> Fx/1(Bx)
  Selector1/1 -> [u]
  [u] -> Saturation6/1
  [Bv] -> Fx/2(Bv)
  Selector6/1 -> [q]
  Bv/1 -> Selector1/1, Selector6/1, [Bv]
  Alpha/1 -> [alpha]
  [alpha] -> Saturation2/1
  dLCG/1 -> [dLCG]
  [dLCG] -> Fx/8(dLCG)
  dmass/1 -> [dMass]
  [dMass] -> Fx/9(dmass)
  Fx/2(Xapp) -> [X_App]
  Fx/3(Xhull) -> [X_Hull]
  Fx/5(X_Hyd) -> [X_Hyd]
  Fx/4(Tout) -> [X_Prop]
  Fx/7(Xstat) -> [X_Stat]
  B_FM/1 -> Selector2/1
  Saturation6/1 -> X'uvwV/2
  Abs/1 -> Xqq/1
  [q] -> Abs/1
  Fx/1(X) -> X/1, [X_Total]
  Saturation2/1 -> X'uvwV/1

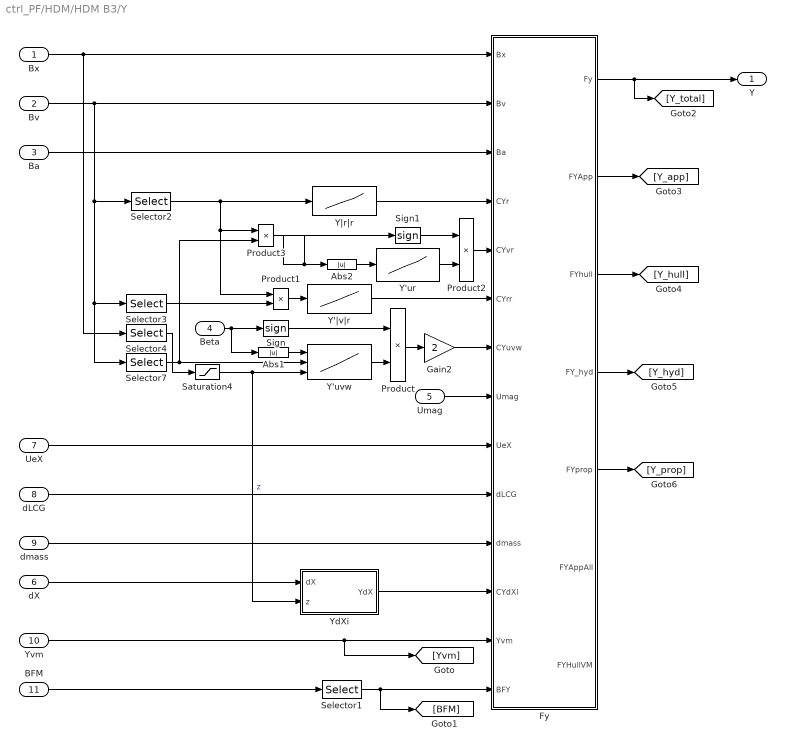
== system ctrl_PF/HDM/HDM B3/Y ==
  Bx : Inport
  Bv : Inport  Port=2
  Ba : Inport  Port=3
  Beta : Inport  Port=4
  Umag : Inport  Port=5
  dX : Inport  Port=6
  UeX : Inport  Port=7
  dLCG : Inport  Port=8
  dmass : Inport  Port=9
  Yvm : Inport  Port=10
  BFM : Inport  Port=11
  Abs1 : Abs  SaturateOnIntegerOverflow=off
  Abs2 : Abs  SaturateOnIntegerOverflow=off
  Fy : MATLAB Function  TreatAsAtomicUnit=on
  Gain2 : Gain  Gain=2
  Product{,1..3} (4 alike) : Product
  Saturation4 : Saturate  UpperLimit=-13.8724  LowerLimit=-35.0624
  Selector1 : Selector  InputPortWidth=6  IndexOptions=Index vector (dialog)  Indices=2  OutputSizes=1
  Selector2 : Selector  InputPortWidth=6  IndexOptions=Index vector (dialog)  Indices=6  OutputSizes=1
  Selector3 : Selector  InputPortWidth=6  IndexOptions=Index vector (dialog)  Indices=2  OutputSizes=1
  Selector4 : Selector  InputPortWidth=6  IndexOptions=Index vector (dialog)  Indices=3  OutputSizes=1
  Selector7 : Selector  InputPortWidth=6  IndexOptions=Index vector (dialog)  Indices=1  OutputSizes=1
  Sign : Signum
  Sign1 : Signum
  Y'ur : Lookup_n-D  NumberOfTableDimensions=1  BreakpointsForDimension1=|  Table=|  InternalRulePriority=Speed  RndMeth=Simplest
      BreakpointsForDimension1=|
      | [0.03999989
      | 0.079999993
      | 0.11999963
      | 0.15999956]
      Table=|
      | [-5.2094E-04
      | -1.0594E-03
      | -1.5649E-03
      | -2.0981E-03]
  Y'uvw : Lookup_n-D  NumberOfTableDimensions=3  BreakpointsForDimension1=|  BreakpointsForDimension2=|  BreakpointsForDimension3=|  Table=|  InternalRulePriority=Speed  RndMeth=Simplest
      BreakpointsForDimension1=|
      | [0
      | 4
      | 8
      | 12]
      BreakpointsForDimension2=|
      | [-5.1444E+00
      | -3.0866E+00
      | -1.5433E+00
      | ]
      Table=|
      | reshape([0.0000000E+00
      | -5.0280621E-03
      | -9.4175348E-03
      | -1.4397458E-02
      | 0.0000000E+00
      | -5.0037454E-03
      | -9.1645405E-03
      | -1.4507402E-02
      | 0.0000000E+00
      | -4.2819107E-03
      | -9.0361786E-03
      | -1.4507235E-02
      | 0.0000000E+00
      | -4.7723270E-03
      | -9.7378407E-03
      | -1.5377541E-02
      | 0.0000000E+00
      | -4.7276301E-03
      | -9.6949815E-03
      | -1.5393721E-02
      | 0.0000000E+00
      | -4.5359209E-03
      | -9.4966039E-03
      | -1.6947859E-02
      | 0.0000000E+00
      | -5.1295007E-03
      | -1.0575377E-02
      | -1.6672924E-02
      | 0.0000000E+00
      | -4.9811404E-03
      | -1.0209461E-02
      | -1.6298327E-02
      | 0.0000000E+00
      | -4.7780219E-03
      | -1.0008968E-02
      | -1.6115181E-02
      | 0.0000000E+00
      | -5.7252015E-03
      | -1.1973447E-02
      | -1.9152812E-02
      | 0.0000000E+00
      | -5.2128737E-03
      | -1.0845978E-02
      | -1.7281669E-02
      | 0.0000000E+00
      | -4.9979037E-03
      | -1.0845685E-02
      | -1.6944141E-02],[4,3,4])
      BreakpointsForDimension3=|
      | [-35.0624 -18.3724 -15.3724 -13.8724
      | ]
      settings: InputPortMap=u0,u1,u2
  Y'|v|r : Lookup_n-D  NumberOfTableDimensions=1  BreakpointsForDimension1=|  Table=|  InternalRulePriority=Speed  RndMeth=Simplest
      BreakpointsForDimension1=|
      | [-0.0015
      | -0.0012
      | -0.0009
      | -0.0006
      | -0.0003
      | -0.0001
      | 0.0001
      | 0.0003
      | 0.0006
      | 0.0009
      | 0.0012
      | 0.0015]
      Table=|
      | [-2.9784E-01
      | -2.6725E-01
      | -2.3292E-01
      | -2.0077E-01
      | -1.1489E-01
      | -7.6673E-03
      | -7.5516E-03
      | -1.1617E-01
      | -2.0077E-01
      | -2.9128E-01
      | -3.5974E-01
      | -4.7839E-01]
  YdXi : Subsystem
  Y|r|r : Lookup_n-D  NumberOfTableDimensions=1  BreakpointsForDimension1=|  Table=|  InternalRulePriority=Speed  RndMeth=Simplest
      BreakpointsForDimension1=|
      | [-0.02
      | -0.015
      | -0.012958963
      | -0.009719222
      | -0.006479482
      | -0.003239741
      | -0.00161987
      | -0.000647948
      | 0.000647948
      | 0.00161987
      | 0.003239741
      | 0.006479482
      | 0.009719222
      | 0.012958963
      | 0.015
      | 0.02
      | ]
      Table=|
      | [3.6478E-03
      | 3.8686E-03
      | 3.4313E-03
      | 4.0790E-03
      | 3.9500E-03
      | 3.6018E-03
      | 3.6796E-03
      | 3.5502E-03
      | 3.4310E-03
      | 3.4872E-03
      | 4.2239E-03
      | 4.0934E-03
      | 3.0314E-03
      | 2.5726E-03
      | 2.9188E-03
      | 2.7740E-03
      | ]
  Y : Outport
  wires:
  Fy/5(FYprop) -> [Y_prop]
  Fy/4(FY_hyd) -> [Y_hyd]
  Fy/3(FYhull) -> [Y_hull]
  Fy/2(FYApp) -> [Y_app]
  YdXi/1(YdX) -> Fy/12(CYdXi)
  Saturation4/1 -> Y'uvw/3, YdXi/2(z)  "z"
  Selector1/1 -> Fy/14(BFY), [BFM]
  BFM/1 -> Selector1/1
  Yvm/1 -> [Yvm], Fy/13(Yvm)
  Gain2/1 -> Fy/7(CYuvw)
  Product/1 -> Gain2/1
  Abs2/1 -> Y'ur/1
  Sign1/1 -> Product2/1
  Product2/1 -> Fy/5(CYvr)
  Abs1/1 -> Y'uvw/1
  Sign/1 -> Product/1
  Y'uvw/1 -> Product/2
  Selector4/1 -> Saturation4/1
  Y'ur/1 -> Product2/2
  Y|r|r/1 -> Fy/4(CYr)
  Fy/1(Fy) -> Y/1, [Y_total]
  Y'|v|r/1 -> Fy/6(CYrr)
  Selector2/1 -> Y|r|r/1, Product3/1, Product1/1
  Product1/1 -> Y'|v|r/1
  Product3/1 -> Abs2/1, Sign1/1
  dX/1 -> YdXi/1(dX)
  dmass/1 -> Fy/11(dmass)
  dLCG/1 -> Fy/10(dLCG)
  Ba/1 -> Fy/3(Ba)
  Selector3/1 -> Product1/2
  UeX/1 -> Fy/9(UeX)
  Bx/1 -> Selector4/1, Fy/1(Bx)
  Umag/1 -> Fy/8(Umag)
  Bv/1 -> Selector7/1, Selector3/1, Selector2/1, Fy/2(Bv)
  Beta/1 -> Abs1/1, Sign/1
  Selector7/1 -> Product3/2, Y'uvw/2

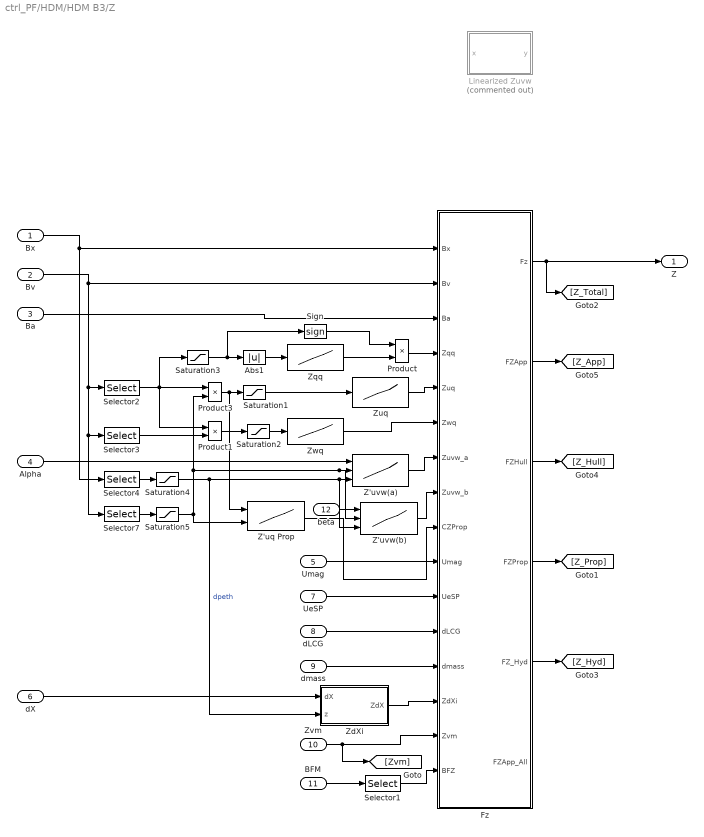
== system ctrl_PF/HDM/HDM B3/Z ==
  Bx : Inport
  Bv : Inport  Port=2
  Ba : Inport  Port=3
  Alpha : Inport  Port=4
  Umag : Inport  Port=5
  dX : Inport  Port=6
  UeSP : Inport  Port=7
  dLCG : Inport  Port=8
  dmass : Inport  Port=9
  Zvm : Inport  Port=10
  BFM : Inport  Port=11
  beta : Inport  Port=12
  Abs1 : Abs  SaturateOnIntegerOverflow=off
  Fz : MATLAB Function  TreatAsAtomicUnit=on
  Linearized Zuvw : MATLAB Function  Commented=on  TreatAsAtomicUnit=on
  Product : Product
  Product1 : Product
  Product3 : Product
  Saturation1 : Saturate  UpperLimit=0.04  LowerLimit=-0.04
  Saturation2 : Saturate  UpperLimit=0.0015  LowerLimit=-0.0015
  Saturation3 : Saturate  UpperLimit=0.02  LowerLimit=-0.02
  Saturation4 : Saturate  UpperLimit=-13.8724  LowerLimit=-35.0624
  Saturation5 : Saturate  UpperLimit=-1.5433E+00  LowerLimit=-5.14444
  Selector1 : Selector  InputPortWidth=6  IndexOptions=Index vector (dialog)  Indices=3  OutputSizes=1
  Selector2 : Selector  InputPortWidth=6  IndexOptions=Index vector (dialog)  Indices=5  OutputSizes=1
  Selector3 : Selector  InputPortWidth=6  IndexOptions=Index vector (dialog)  Indices=3  OutputSizes=1
  Selector4 : Selector  InputPortWidth=6  IndexOptions=Index vector (dialog)  Indices=3  OutputSizes=1
  Selector7 : Selector  InputPortWidth=6  IndexOptions=Index vector (dialog)  Indices=1  OutputSizes=1
  Sign : Signum
  Z'uq Prop : Lookup_n-D  BreakpointsForDimension1=|  BreakpointsForDimension2=[-7.71666 -5.14444 -3.086664 -1.543332]  Table=|  InternalRulePriority=Speed  RndMeth=Simplest
      BreakpointsForDimension1=|
      | [-2.0E-01
      | -1.5E-01
      | -1.0E-01
      | -5.0E-02
      | 0.0E+00
      | 5.0E-02
      | 1.0E-01
      | 1.5E-01
      | 2.0E-01
      | ]
      Table=|
      | reshape([1.3913E-04
      | 1.0452E-04
      | 6.9900E-05
      | 3.5283E-05
      | 6.6700E-07
      | -3.3949E-05
      | -6.8566E-05
      | -1.0318E-04
      | -1.3780E-04
      | 2.8914E-04
      | 2.1702E-04
      | 1.4490E-04
      | 7.2785E-05
      | 6.6700E-07
      | -7.1451E-05
      | -1.4357E-04
      | -2.1569E-04
      | -2.8780E-04
      | 1.1606E-04
      | 8.7208E-05
      | 5.8361E-05
      | 2.9514E-05
      | 6.6700E-07
      | -2.8180E-05
      | -5.7027E-05
      | -8.5874E-05
      | -1.1472E-04
      | 1.1606E-04
      | 8.7208E-05
      | 5.8361E-05
      | 2.9514E-05
      | 6.6700E-07
      | -2.8180E-05
      | -5.7027E-05
      | -8.5874E-05
      | -1.1472E-04],[9,4])
      settings: InputPortMap=u0,u1
  Z'uvw(a) : Lookup_n-D  NumberOfTableDimensions=3  BreakpointsForDimension1=|  BreakpointsForDimension2=|  BreakpointsForDimension3=|  Table=|  InternalRulePriority=Speed  RndMeth=Simplest
      BreakpointsForDimension1=|
      | [-12
      | -8
      | -4
      | 0
      | 4
      | 8
      | 12]
      BreakpointsForDimension2=|
      | [-5.1444E+00
      | -3.0866E+00
      | -1.5433E+00
      | ]
      Table=|
      | reshape([-3.82587E-03
      | -2.42543E-03
      | -1.05453E-03
      | 1.94202E-04
      | 1.48991E-03
      | 3.04047E-03
      | 4.14104E-03
      | -3.76348E-03
      | -2.38508E-03
      | -9.82619E-04
      | 1.94202E-04
      | 1.47560E-03
      | 3.02863E-03
      | 4.06663E-03
      | -3.75964E-03
      | -2.29001E-03
      | -8.34074E-04
      | 1.94202E-04
      | 1.38956E-03
      | 2.91153E-03
      | 4.15251E-03
      | -3.11218E-03
      | -1.80502E-03
      | -4.97855E-04
      | 8.09305E-04
      | 2.11647E-03
      | 3.42363E-03
      | 4.73079E-03
      | -2.62573E-03
      | -1.48072E-03
      | -3.35708E-04
      | 8.09305E-04
      | 1.95432E-03
      | 3.09933E-03
      | 4.24434E-03
      | -2.06413E-03
      | -1.10632E-03
      | -1.48507E-04
      | 8.09305E-04
      | 1.76712E-03
      | 2.72493E-03
      | 3.68274E-03
      | -3.09997E-03
      | -1.76300E-03
      | -4.26025E-04
      | 9.10947E-04
      | 2.24792E-03
      | 3.58489E-03
      | 4.92186E-03
      | -2.49055E-03
      | -1.35672E-03
      | -2.22886E-04
      | 9.10947E-04
      | 2.04478E-03
      | 3.17861E-03
      | 4.31245E-03
      | -2.64104E-03
      | -1.45704E-03
      | -2.73048E-04
      | 9.10947E-04
      | 2.09494E-03
      | 3.27894E-03
      | 4.46293E-03
      | -0.003059752
      | -0.001711935
      | -0.000364117
      | 0.0009837
      | 0.002331518
      | 0.003679335
      | 0.005027153
      | -0.002351082
      | -0.0012256
      | -0.000100118
      | 0.0009837
      | 0.002109182
      | 0.003234664
      | 0.004360146
      | -0.001725739
      | -0.000822593
      | 8.05539E-05
      | 0.0009837
      | 0.001886847
      | 0.002789993
      | 0.00369314],[7,3,4])
      BreakpointsForDimension3=|
      | [-35.0624 -18.3724 -15.3724 -13.8724
      | ]
      settings: InputPortMap=u0,u1,u2
  Z'uvw(b) : Lookup_n-D  NumberOfTableDimensions=3  BreakpointsForDimension1=|  BreakpointsForDimension2=|  BreakpointsForDimension3=|  Table=|  InternalRulePriority=Speed  RndMeth=Simplest
      BreakpointsForDimension1=|
      | [0
      | 4
      | 8
      | 12]
      BreakpointsForDimension2=|
      | [-5.1444E+00
      | -3.0866E+00
      | -1.5433E+00
      | ]
      Table=|
      | reshape([0.0000000E+00
      | -5.9986916E-04
      | -2.7503348E-03
      | -5.0777589E-03
      | 0.0000000E+00
      | -6.0654884E-04
      | -2.4512564E-03
      | -5.2464901E-03
      | 0.0000000E+00
      | -7.6137528E-04
      | -2.4084463E-03
      | -5.2118678E-03
      | 0.0000000E+00
      | -8.2427914E-04
      | -2.5250249E-03
      | -5.3103563E-03
      | 0.0000000E+00
      | -8.1036019E-04
      | -2.5315266E-03
      | -5.5141459E-03
      | 0.0000000E+00
      | -7.9799041E-04
      | -2.5595242E-03
      | -5.2319004E-03
      | 0.0000000E+00
      | -8.6989011E-04
      | -2.5865820E-03
      | -5.6151595E-03
      | 0.0000000E+00
      | -8.4361582E-04
      | -2.6124115E-03
      | -5.7143353E-03
      | 0.0000000E+00
      | -8.2567611E-04
      | -2.6088331E-03
      | -5.6150660E-03
      | 0.0000000E+00
      | -9.1003224E-04
      | -2.7683191E-03
      | -6.0189061E-03
      | 0.0000000E+00
      | -8.4211433E-04
      | -2.5899187E-03
      | -5.7497784E-03
      | 0.0000000E+00
      | -8.2014014E-04
      | -2.4092466E-03
      | -5.6643347E-03],[4,3,4])
      BreakpointsForDimension3=|
      | [-35.0624 -18.3724 -15.3724 -13.8724
      | ]
      settings: InputPortMap=u0,u1,u2
  ZdXi : Subsystem
  Zqq : Lookup_n-D  NumberOfTableDimensions=1  BreakpointsForDimension1=|  Table=|  InternalRulePriority=Speed  RndMeth=Simplest
      BreakpointsForDimension1=|
      | [0.000127901
      | 0.000383704
      | 0.000639507
      | 0.001279013
      | 0.002558026
      | ]
      Table=|
      | [-1.5611E-03
      | -1.0379E-04
      | 3.9238E-05
      | 1.1475E-04
      | 1.3579E-04
      | ]
  Zuq : Lookup_n-D  NumberOfTableDimensions=1  BreakpointsForDimension1=|  Table=|  InternalRulePriority=Speed  RndMeth=Simplest
      BreakpointsForDimension1=|
      | [-0.04
      | -0.03
      | -0.02
      | -0.01
      | -0.005
      | -0.002
      | 0.002
      | 0.005
      | 0.01
      | 0.02
      | 0.03
      | 0.04
      | ]
      Table=|
      | [-9.8908E-03
      | -9.0784E-03
      | -8.9566E-03
      | -1.0733E-02
      | -1.4141E-02
      | -2.4189E-02
      | -6.5605E-03
      | -7.1594E-03
      | -7.6366E-03
      | -7.9008E-03
      | -6.1794E-03
      | -6.1029E-03
      | ]
  Zwq : Lookup_n-D  NumberOfTableDimensions=1  BreakpointsForDimension1=|  Table=|  InternalRulePriority=Speed  RndMeth=Simplest
      BreakpointsForDimension1=|
      | [-0.0015
      | -0.0012
      | -0.0009
      | -0.0006
      | -0.0003
      | -0.0001
      | 0.0001
      | 0.0003
      | 0.0006
      | 0.0009
      | 0.0012
      | 0.0015]
      Table=|
      | [-2.9784E-01
      | -2.6725E-01
      | -2.3292E-01
      | -2.0077E-01
      | -1.1489E-01
      | -7.6673E-03
      | -7.5516E-03
      | -1.1617E-01
      | -2.0077E-01
      | -2.9128E-01
      | -3.5974E-01
      | -4.7839E-01]
  Z : Outport
  wires:
  beta/1 -> Z'uvw(b)/1
  Z'uvw(b)/1 -> Fz/8(Zuvw_b)
  Product/1 -> Fz/4(Zqq)
  Sign/1 -> Product/1
  Abs1/1 -> Zqq/1
  Selector7/1 -> Saturation5/1
  Saturation5/1 -> Z'uq Prop/2, Z'uvw(b)/2, Z'uvw(a)/2, Product3/2
  Saturation4/1 -> ZdXi/2(z), Z'uvw(a)/3, Z'uvw(b)/3  "dpeth"
  Fz/5(FZ_Hyd) -> [Z_Hyd]
  Fz/4(FZProp) -> [Z_Prop]
  Fz/3(FZHull) -> [Z_Hull]
  Fz/2(FZApp) -> [Z_App]
  ZdXi/1(ZdX) -> Fz/14(ZdXi)
  Selector1/1 -> Fz/16(BFZ)
  BFM/1 -> Selector1/1
  Z'uvw(a)/1 -> Fz/7(Zuvw_a)
  Zqq/1 -> Product/2
  Z'uq Prop/1 -> Fz/9(CZProp)
  Zwq/1 -> Fz/6(Zwq)
  Selector2/1 -> Saturation3/1, Product1/1, Product3/1
  Alpha/1 -> Z'uvw(a)/1
  Bv/1 -> Selector7/1, Selector3/1, Selector2/1, Fz/2(Bv)
  Umag/1 -> Fz/10(Umag)
  Bx/1 -> Selector4/1, Fz/1(Bx)
  Product3/1 -> Z'uq Prop/1, Saturation1/1
  UeSP/1 -> Fz/11(UeSP)
  Selector3/1 -> Product1/2
  Product1/1 -> Saturation2/1
  dLCG/1 -> Fz/12(dLCG)
  dmass/1 -> Fz/13(dmass)
  dX/1 -> ZdXi/1(dX)
  Saturation1/1 -> Zuq/1
  Saturation2/1 -> Zwq/1
  Saturation3/1 -> Sign/1, Abs1/1
  Fz/1(Fz) -> [Z_Total], Z/1
  Zuq/1 -> Fz/5(Zuq)
  Ba/1 -> Fz/3(Ba)
  Zvm/1 -> [Zvm], Fz/15(Zvm)
  Selector4/1 -> Saturation4/1

== system ctrl_PF/HDM/Integration and Coord. Transfrom/Coordinate Transform ==
  Bv : Inport
  Integrator : Integrator  InitialCondition=Bx_0
  MATLAB Function2 : MATLAB Function  TreatAsAtomicUnit=on
  X_earth : Outport  VectorParamsAs1DForOutWhenUnconnected=off
  wires:
  MATLAB Function2/1(out) -> Integrator/1
  Bv/1 -> MATLAB Function2/2(Bv)
  Integrator/1 -> X_earth/1, MATLAB Function2/1(Bx)

== system ctrl_PF/HDM/Integration and Coord. Transfrom/Rigid Body Motion ==
  F_hyd : Inport
  Bx : Inport  Port=2
  Demux : Demux  Outputs=6
  Demux1 : Demux  Outputs=6
  Demux2 : Demux  Outputs=5
  Gain2 : Gain
  Integrator : Integrator  InitialCondition=Bv_0
  MATLAB Function2 : MATLAB Function  TreatAsAtomicUnit=on
  Memory1 : Memory  InitialCondition=Ba_0
  Mux1 : Mux  Inputs=6
  Mux2 : Mux  Inputs=5
  Bv : Outport  VectorParamsAs1DForOutWhenUnconnected=off
  Ba : Outport  Port=2  VectorParamsAs1DForOutWhenUnconnected=off
  wires:
  Mux1/1 -> Bv/1
  Gain2/1 -> Demux2/1
  Demux1/2 -> Mux2/1
  Demux1/4 -> Mux2/3
  Demux1/6 -> Mux2/5
  Demux1/5 -> Mux2/4
  Demux2/1 -> Mux1/2
  Demux1/1 -> Mux1/1
  Demux2/4 -> Mux1/5
  Demux2/2 -> Mux1/3
  Demux2/5 -> Mux1/6
  Mux2/1 -> Gain2/1
  Demux1/3 -> Mux2/2
  Demux2/3 -> Mux1/4
  F_hyd/1 -> Demux/1
  Demux/6 -> MATLAB Function2/6(N)
  Demux/5 -> MATLAB Function2/5(M)
  Demux/4 -> MATLAB Function2/4(K)
  Demux/3 -> MATLAB Function2/3(Z)
  Demux/2 -> MATLAB Function2/2(Y)
  Demux/1 -> MATLAB Function2/1(X)
  Memory1/1 -> Ba/1
  Integrator/1 -> Demux1/1, MATLAB Function2/8(bv)
  MATLAB Function2/1(out) -> Memory1/1, Integrator/1
  Bx/1 -> MATLAB Function2/7(bx)

== system ctrl_PF/HDM/actuator saturation/  ==
  "dX " : Inport
  Constant{,3,5,7,9} (5 alike) : Constant  Value=7.11
  Constant{2,4,6,8,10} (5 alike) : Constant  Value=-7.11
  Demux3 : Demux  Outputs=5
  I-Pitch{1..5} (5 alike) : Gain
  Max Deflection{,1..4} (5 alike) : Saturate  UpperLimit=30  LowerLimit=-30
  Mux : Mux  Inputs=5
  Rate Limiter Dynamic{,1..4} (5 alike) : simulink/Discontinuities/Rate Limiter Dynamic
  Scope : Scope  NumInputPorts=5
  dX : Outport
  wires:
  Rate Limiter Dynamic3/1 -> Max Deflection3/1
  Mux/1 -> dX/1
  Constant7/1 -> Rate Limiter Dynamic3/1
  Max Deflection4/1 -> I-Pitch5/1  "dV"
  Constant8/1 -> Rate Limiter Dynamic3/3
  "dX "/1 -> Demux3/1
  Max Deflection3/1 -> I-Pitch4/1  "dV"
  Constant5/1 -> Rate Limiter Dynamic2/1
  Max Deflection1/1 -> I-Pitch1/1  "dV"
  Rate Limiter Dynamic2/1 -> Max Deflection2/1
  Constant/1 -> Rate Limiter Dynamic/1
  Rate Limiter Dynamic1/1 -> Max Deflection1/1
  Constant6/1 -> Rate Limiter Dynamic2/3
  I-Pitch4/1 -> Mux/4, Scope/4
  I-Pitch3/1 -> Mux/1, Scope/1
  Constant4/1 -> Rate Limiter Dynamic1/3
  I-Pitch1/1 -> Mux/2, Scope/2
  Max Deflection2/1 -> I-Pitch2/1  "dV"
  Rate Limiter Dynamic4/1 -> Max Deflection4/1
  I-Pitch5/1 -> Mux/5, Scope/5
  Rate Limiter Dynamic/1 -> Max Deflection/1
  Constant10/1 -> Rate Limiter Dynamic4/3
  Demux3/2 -> Rate Limiter Dynamic1/2
  Demux3/4 -> Rate Limiter Dynamic3/2
  Constant3/1 -> Rate Limiter Dynamic1/1
  Demux3/5 -> Rate Limiter Dynamic4/2
  Demux3/3 -> Rate Limiter Dynamic2/2
  Max Deflection/1 -> I-Pitch3/1  "dV"
  Demux3/1 -> Rate Limiter Dynamic/2
  Constant9/1 -> Rate Limiter Dynamic4/1
  Constant2/1 -> Rate Limiter Dynamic/3
  I-Pitch2/1 -> Mux/3, Scope/3

== system ctrl_PF/HDM/actuator saturation/    ==
  "n " : Inport
  Rate Limiter Dynamic : simulink/Discontinuities/Rate Limiter Dynamic
  Rate Max : Constant  Value=14.65
  Rate Min : Constant  Value=-14.65
  Saturation6 : Saturate  UpperLimit=10  LowerLimit=0.01
  n : Outport
  wires:
  Saturation6/1 -> n/1
  Rate Max/1 -> Rate Limiter Dynamic/1
  Rate Limiter Dynamic/1 -> Saturation6/1
  Rate Min/1 -> Rate Limiter Dynamic/3
  "n "/1 -> Rate Limiter Dynamic/2
